simulink model "untitled1"  (R2022b)
settings: Solver=FixedStepDiscrete  StartTime=0.0  StopTime=10.0  FixedStep=Ts  RelTol=1e-3
values from neighbouring files (symbols this model uses):
  Ad = exp(A*Ts)    [O1sys0.m]    (also in kalmf_rep.m = exp(-a*Ts); noise_01.m = exp(-a * Ts); noise_02.m = expm(sys.A * Ts))
  H = h    [O1sys0.m]    (also in kalmf_rep.m = 0)
  M = [0 P;1 0;0 P]    [SampledDataSystem.m]
  R = .5    (= 0.5)    [O1sys0.m]    (also in kalmf_rep.m = 0.4)
  Ts = .02    (= 0.02)    [O1sys0.m]    (also in SampledDataSystem.m = 0.1; kalmf_rep.m; noise_01.m = 0.01; noise_02.m = 0.01)
  x0 = 3    [O1sys0.m]
undefined symbols (not defined in the file or in its folder): Discrete, Time, Tv, Tw
libraries: ctrlSharedLib x1
settings Model: Creator=hp_desktop  LastModifiedBy=hp_desktop

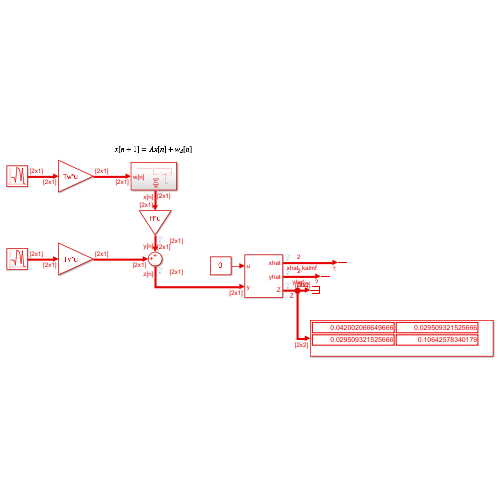
[thumbnail: Simulink's stored preview of the top-level diagram]
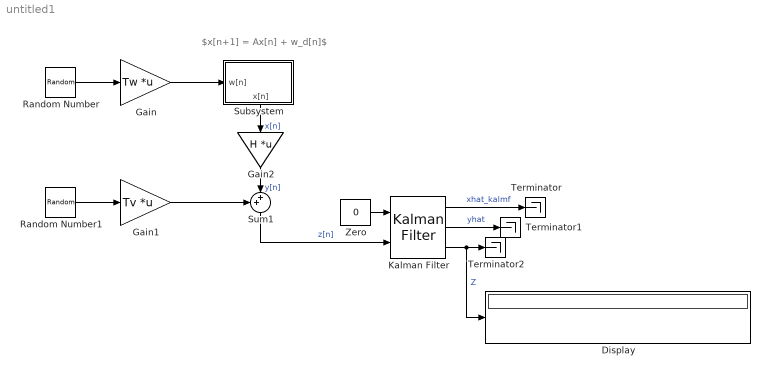
== system untitled1 ==
  note: $x[n+1] = Ax[n] + w_d[n]$
  Display : Display
  Gain : Gain  Gain=Tw  Multiplication=Matrix(K*u)
  Gain1 : Gain  Gain=Tv  Multiplication=Matrix(K*u)
  Gain2 : Gain  Gain=H  Multiplication=Matrix(K*u)
  Kalman Filter : ctrlSharedLib/Kalman Filter  TimeDomain=Discrete-Time  UseCurrentEstimator=on  ModelSource=Individual A, B, C, D matrices  ModelSourceVariable=ss(0.95,1,1,0,1)  A=Ad  B=[0;0]  C=H  D=zeros(M,1)  NumberOfStates=1  NumberOfInputs=1  NumberOfOutputs=1  InitialEstimateSource=Dialog  X0=x0  P0=10  UseK=off  UseGH=off  NumberOfProcessNoiseInputs=1  G=1  TimeInvariantG=on  H=0  TimeInvariantH=on  Q=Qd  TimeInvariantQ=on  R=R  TimeInvariantR=on  N=0  TimeInvariantN=on  AddInputPort=on  AddEnablePort=off  OutputEstimatedY=on  OutputP=on  Ts=-1
  Random Number : RandomNumber  Seed=[0;1e3]  SampleTime=Ts  VectorParams1D=off
  Random Number1 : RandomNumber  Seed=randi(1e4,M,1) + 1e3  SampleTime=Ts  VectorParams1D=off
  Subsystem : Subsystem
      settings: PortSchema="{\"entries\":[{\"content\":{\"sides\":[{\"content\":{\"connectorIds\":[\"In1\"]},\"type\":\"ConnectorPlacement.EquallySpacedRectSide\",\"uuid\":\"ef2e77e5-091a-4ff0-8195-284a768bf301\"},{\"content\":{\"connectorIds\":[],\"side\":\"RIGHT\"},\"type\":\"ConnectorPlacement.EquallySpacedRectSide\",\"uuid\":\"8fd17047-c7ad-4e52-8674-6e8fe37ffb09\"},{\"content\":{\"connectorIds\":[],\"side\":\"TOP\"},\"type\":\"ConnectorPlacement.EquallySpacedRectSide\",\"uuid\":\"ac4ef6ef-d465-4745-a23e-471090b17812\"},{\"content\":{\"connectorIds\":[\"Out1\"],\"side\":\"BOTTOM\"},\"type\":\"ConnectorPlacement.EquallySpacedRectSide\",\"uuid\":\"58061811-e53b-4936-b707-bae3455a4e49\"}]},\"type\":\"ConnectorPlacement.EquallySpacedConnector\",\"uuid\":\"082ec2b0-1d9b-4f43-a721-d8e0d8a60c1d\"}],\"packageUris\":[\"http://schema.mathworks.com/mf0/Connector/R2020b\"],\"version\":\"1.0\"}"
  Sum1 : Sum  Inputs=++|
  Terminator : Terminator
  Terminator1 : Terminator
  Terminator2 : Terminator
  Zero : Constant  Value=0  OutDataTypeStr=Inherit: Inherit via back propagation  SampleTime=-1
  wires:
  Random Number/1 -> Gain/1
  Gain/1 -> Subsystem/1(w[n])
  Subsystem/1(x[n]) -> Gain2/1  "x[n]"
  Gain1/1 -> Sum1/1
  Random Number1/1 -> Gain1/1
  Zero/1 -> Kalman Filter/1
  Kalman Filter/1 -> Terminator/1  "xhat_kalmf"
  Sum1/1 -> Kalman Filter/2  "z[n]"
  Gain2/1 -> Sum1/2  "y[n]"
  Kalman Filter/2 -> Terminator1/1  "yhat"
  Kalman Filter/3 -> Display/1, Terminator2/1  "Z"

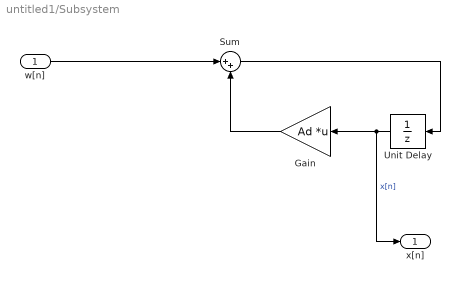
== system untitled1/Subsystem ==
  w[n] : Inport
  Gain : Gain  Gain=Ad  Multiplication=Matrix(K*u)
  Sum : Sum  Inputs=|++
  Unit Delay : UnitDelay  InitialCondition=x0  SampleTime=-1  HasFrameUpgradeWarning=on
  x[n] : Outport
  wires:
  Sum/1 -> Unit Delay/1
  w[n]/1 -> Sum/1
  Unit Delay/1 -> x[n]/1, Gain/1  "x[n]"
  Gain/1 -> Sum/2
